simulink model "simula_levitador_non_linear"  (R2024b)
settings: Solver=ode15s  StartTime=0.0  StopTime=10.0  RelTol=1e-6
values from neighbouring files (symbols this model uses):
  a = 6.72e-3    (= 0.00672)    [analise_estabilidade_levitador.m]    (also in analise_estabilidade_levitador_certo.m; run_simulator_levitador_magnetic.m)
  c1 = -1.7361e3    (= -1736.1)    [analise_estabilidade_levitador.m]    (also in analise_estabilidade_levitador_certo.m; run_simulator_levitador_magnetic.m)
  g = 9.81    [analise_estabilidade_levitador.m]    (also in analise_estabilidade_levitador_certo.m; run_simulator_levitador_magnetic.m)
  h0 = 10e-3    (= 0.01)    [analise_estabilidade_levitador_certo.m]    (also in run_simulator_levitador_magnetic.m)
  he = 4.5e-3    (= 0.0045)    [analise_estabilidade_levitador.m]    (also in analise_estabilidade_levitador_certo.m; run_simulator_levitador_magnetic.m)
  i0 = 0.39    [analise_estabilidade_levitador_certo.m]    (also in run_simulator_levitador_magnetic.m)
  ka = 2.1    [analise_estabilidade_levitador.m]    (also in analise_estabilidade_levitador_certo.m; run_simulator_levitador_magnetic.m)
  kp = 1    [analise_estabilidade_levitador.m]    (also in analise_estabilidade_levitador_certo.m = 0.4; run_simulator_levitador_magnetic.m)
  L0 = 24.9e-3    (= 0.0249)    [analise_estabilidade_levitador.m]    (also in analise_estabilidade_levitador_certo.m; run_simulator_levitador_magnetic.m)
  Le = 520e-3    (= 0.52)    [analise_estabilidade_levitador.m]    (also in analise_estabilidade_levitador_certo.m; run_simulator_levitador_magnetic.m)
  m = 22.6e-3    (= 0.0226)    [analise_estabilidade_levitador.m]    (also in analise_estabilidade_levitador_certo.m; run_simulator_levitador_magnetic.m)
  R = 21    [analise_estabilidade_levitador.m]    (also in analise_estabilidade_levitador_certo.m; run_simulator_levitador_magnetic.m)
  tp = 0.004    [analise_estabilidade_levitador.m]    (also in analise_estabilidade_levitador_certo.m; run_simulator_levitador_magnetic.m)
  tz = 0.04    [analise_estabilidade_levitador.m]    (also in analise_estabilidade_levitador_certo.m; run_simulator_levitador_magnetic.m)
  v0 = 0    [analise_estabilidade_levitador_certo.m]    (also in run_simulator_levitador_magnetic.m)
  ve = R*ie/ka    [analise_estabilidade_levitador.m]    (also in analise_estabilidade_levitador_certo.m; run_simulator_levitador_magnetic.m)
settings Model: Creator=engma  LastModifiedBy=engma

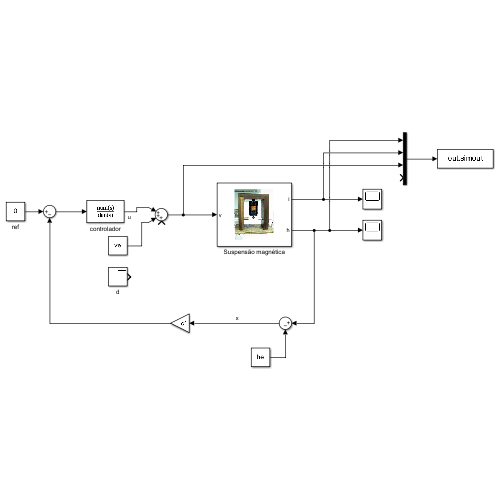
[thumbnail: Simulink's stored preview of the top-level diagram]
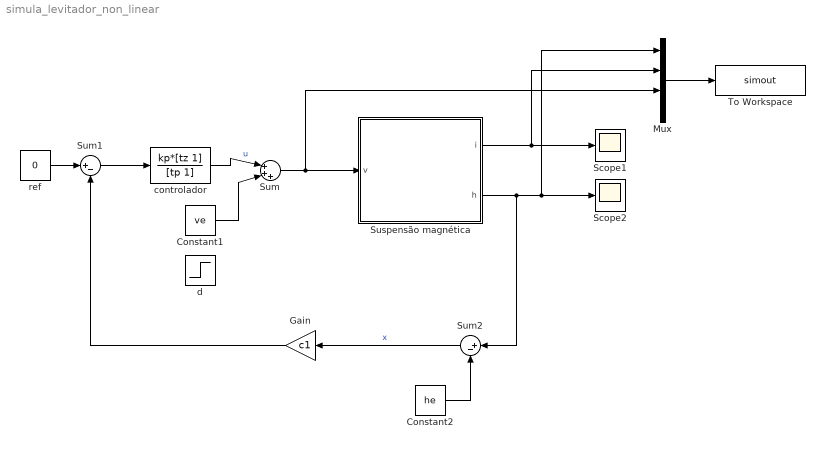
== system simula_levitador_non_linear ==
  Constant1 : Constant  Value=ve
  Constant2 : Constant  Value=he
  Gain : Gain  Gain=c1
  Mux : Mux
  Scope1 : Scope
  Scope2 : Scope
  Sum : Sum  Inputs=|+++
  Sum1 : Sum  Inputs=|+-
  Sum2 : Sum  Inputs=|+-
  Suspensão magnética : Subsystem
      mask Display: image('levitador.png', [10,10,10,10,100,100]);
  To Workspace : ToWorkspace  VariableName=simout  SaveFormat=Structure With Time  SampleTime=-1
  controlador : TransferFcn  Numerator=kp*[tz 1]  Denominator=[tp 1]
  d : Step  After=0.1  SampleTime=0
  ref : Constant  Value=0
  wires:
  Suspensão magnética/1(i) -> Mux/2, Scope1/1
  Suspensão magnética/2(h) -> Sum2/1, Mux/1, Scope2/1
  Sum/1 -> Mux/3, Suspensão magnética/1(v)
  Constant1/1 -> Sum/2
  Sum2/1 -> Gain/1  "x"
  Constant2/1 -> Sum2/2
  controlador/1 -> Sum/1  "u"
  Mux/1 -> To Workspace/1
  ref/1 -> Sum1/1
  Gain/1 -> Sum1/2
  Sum1/1 -> controlador/1

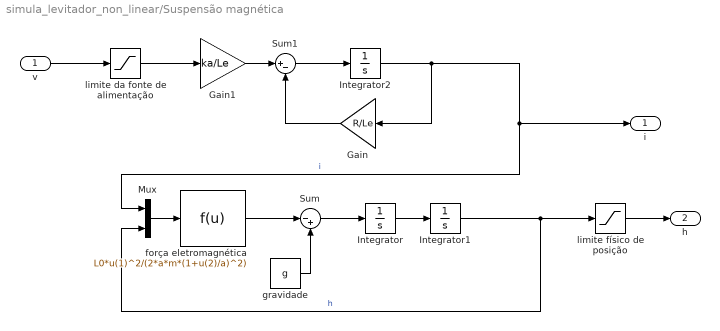
== system simula_levitador_non_linear/Suspensão magnética ==
  v : Inport
  Gain : Gain  Gain=R/Le
  Gain1 : Gain  Gain=ka/Le
  Integrator : Integrator  InitialCondition=v0
  Integrator1 : Integrator  InitialCondition=h0
  Integrator2 : Integrator  InitialCondition=i0
  Mux : Mux  Inputs=2
  Sum : Sum  Inputs=|-+
  Sum1 : Sum  Inputs=|+-
  força eletromagnética : Fcn  Expr=L0*u(1)^2/(2*a*m*(1+u(2)/a)^2)
  gravidade : Constant  Value=g
  limite da fonte de alimentação : Saturate  UpperLimit=24  LowerLimit=-24
  limite físico de posição : Saturate  UpperLimit=1  LowerLimit=0
  i : Outport
  h : Outport  Port=2
  wires:
  Integrator1/1 -> limite físico de posição/1, Mux/2  "h"
  Gain1/1 -> Sum1/1
  gravidade/1 -> Sum/2
  Gain/1 -> Sum1/2
  Integrator2/1 -> i/1, Mux/1, Gain/1  "i"
  Sum/1 -> Integrator/1
  força eletromagnética/1 -> Sum/1
  Sum1/1 -> Integrator2/1
  Integrator/1 -> Integrator1/1
  Mux/1 -> força eletromagnética/1
  v/1 -> limite da fonte de alimentação/1
  limite da fonte de alimentação/1 -> Gain1/1
  limite físico de posição/1 -> h/1
